simulink model "SmallScaleFilter"  (R2023b)
settings: Solver=FixedStepDiscrete  StartTime=0.0  StopTime=inf  RelTol=1e-3
libraries: simulink x1
settings Model: Creator=madeline  LastModifiedBy=madeline

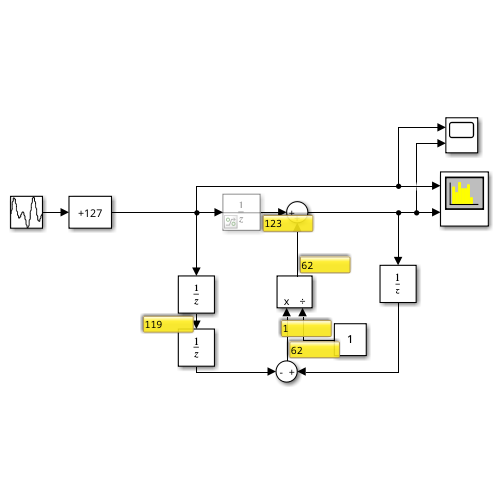
[thumbnail: Simulink's stored preview of the top-level diagram]
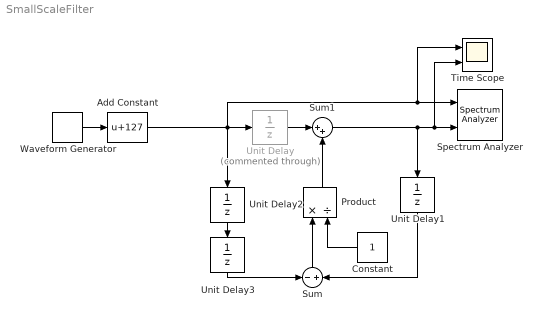
== system SmallScaleFilter ==
  Add Constant : Bias  Bias=127  SaturateOnIntegerOverflow=off
  Constant : Constant  OutDataTypeStr=uint8
  Product : Product  Inputs=*/  OutDataTypeStr=Inherit: Same as first input
  Spectrum Analyzer : SpectrumAnalyzer  NumInputPorts=2  WindowPosition=[140.000000,543.000000,800.000000,500.000000,]  ScopeFrameLocation=window  PlotAsTwoSidedSpectrum=off  FrequencyScale=Log  Span=5  CenterFrequency=2.5  StartFrequency=0  StopFrequency=5  YLimits=[-3.49779931,84.65733127]  SelectedToolstripTab=spectrumAnalyzerToolstrip.spectrumTab
  Sum : Sum  Inputs=-|+
  Sum1 : Sum  Inputs=|++
  Time Scope : Scope  NumInputPorts=2
  Unit Delay : UnitDelay  Commented=through  SampleTime=-1  HasFrameUpgradeWarning=on
  Unit Delay1 : UnitDelay  SampleTime=-1  HasFrameUpgradeWarning=on
  Unit Delay2 : UnitDelay  SampleTime=-1  HasFrameUpgradeWarning=on
  Unit Delay3 : UnitDelay  SampleTime=-1  HasFrameUpgradeWarning=on
  Waveform Generator : simulink/Sources/Waveform Generator  OutMin=[]  OutMax=[]  OutDataTypeStr=uint8  SelectedSignal=1  Signals=gaussian('Mean',0,'Variance', 127, 'Seed',1)#sin(127,1000,0)  BlockNames=MultiportSwitch_e6899b5ed281472#MultiportSwitch_c717f1cb9880493  SampleTime=0.00005
  wires:
  Unit Delay1/1 -> Sum/2
  Sum1/1 -> Time Scope/2, Spectrum Analyzer/2, Unit Delay1/1
  Waveform Generator/1 -> Add Constant/1
  Add Constant/1 -> Unit Delay2/1, Unit Delay/1, Time Scope/1, Spectrum Analyzer/1
  Sum/1 -> Product/1
  Constant/1 -> Product/2
  Unit Delay/1 -> Sum1/1
  Product/1 -> Sum1/2
  Unit Delay2/1 -> Unit Delay3/1
  Unit Delay3/1 -> Sum/1
